simulink model "Mbase4_sim"  (R2014a)
settings: Solver=ode45  StartTime=0.0  StopTime=30  RelTol=1e-3
libraries: arduino_io_lib x5, simulink x1
settings Model: Creator=omar_  LastModifiedBy=omar_

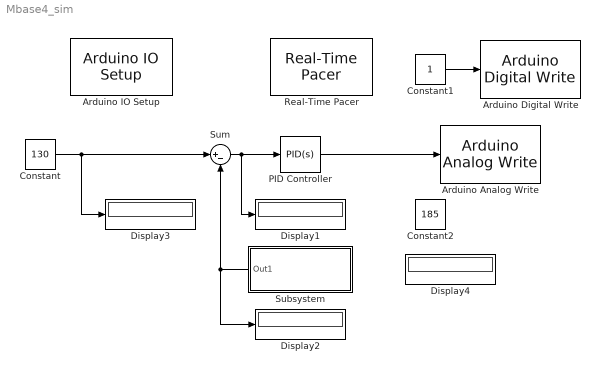
== system Mbase4_sim ==
  Arduino Analog Write : arduino_io_lib/Arduino Analog Write  arduinoVar=Temporary arduino variable: Arduino1  arduinoPin=5  T=0.2
  Arduino Digital Write : arduino_io_lib/Arduino Digital Write  arduinoVar=Temporary arduino variable: Arduino1  arduinoPin=6  T=0.2
  Arduino IO Setup : arduino_io_lib/Arduino IO Setup  Priority=3  arduinoVar=Temporary arduino variable: Arduino1  workspaceVarName=a  comPort=COM3
  Constant : Constant  Value=130
  Constant1 : Constant
  Constant2 : Constant  Value=185
  Display{1..4} (4 alike) : Display
  PID Controller : simulink/Continuous/PID Controller  Controller=PID  TimeDomain=Continuous-time  SampleTime=1  IntegratorMethod=Forward Euler  FilterMethod=Forward Euler  Form=Parallel  P=0.146995673261305  I=0.922603334081805  D=0  N=100  InitialConditionSource=internal  InitialConditionForIntegrator=0  InitialConditionForFilter=0  ExternalReset=none  LimitOutput=off  UpperSaturationLimit=inf  LowerSaturationLimit=-inf  LinearizeAsGain=on  AntiWindupMode=none  Kb=1  TrackingMode=off  Kt=1  PParamMin=[]  PParamMax=[]  IParamMin=[]  IParamMax=[]  DParamMin=[]  DParamMax=[]  NParamMin=[]  NParamMax=[]  KbParamMin=[]  KbParamMax=[]  KtParamMin=[]  KtParamMax=[]  POutMin=[]  POutMax=[]  IOutMin=[]  IOutMax=[]  DOutMin=[]  DOutMax=[]  NOutMin=[]  NOutMax=[]  KbOutMin=[]  KbOutMax=[]  KtOutMin=[]  KtOutMax=[]  IntegratorOutMin=[]  IntegratorOutMax=[]  FilterOutMin=[]  FilterOutMax=[]  SumOutMin=[]  SumOutMax=[]  SumI1OutMin=[]  SumI1OutMax=[]  SumI2OutMin=[]  SumI2OutMax=[]  SumI3OutMin=[]  SumI3OutMax=[]  SumDOutMin=[]  SumDOutMax=[]  SaturationOutMin=[]  SaturationOutMax=[]  IntegratorContinuousStateAttributes=''  IntegratorStateMustResolveToSignalObject=off  IntegratorRTWStateStorageClass=Auto  FilterContinuousStateAttributes=''  FilterStateMustResolveToSignalObject=off  FilterRTWStateStorageClass=Auto
  Real-Time Pacer : arduino_io_lib/Real-Time Pacer  simTimePerRealTime=1
  Subsystem : Subsystem
  Sum : Sum  Inputs=|+-
  wires:
  Constant/1 -> Sum/1, Display3/1
  Sum/1 -> PID Controller/1, Display1/1
  Subsystem/1(Out1) -> Display2/1, Sum/2
  PID Controller/1 -> Arduino Analog Write/1
  Constant1/1 -> Arduino Digital Write/1

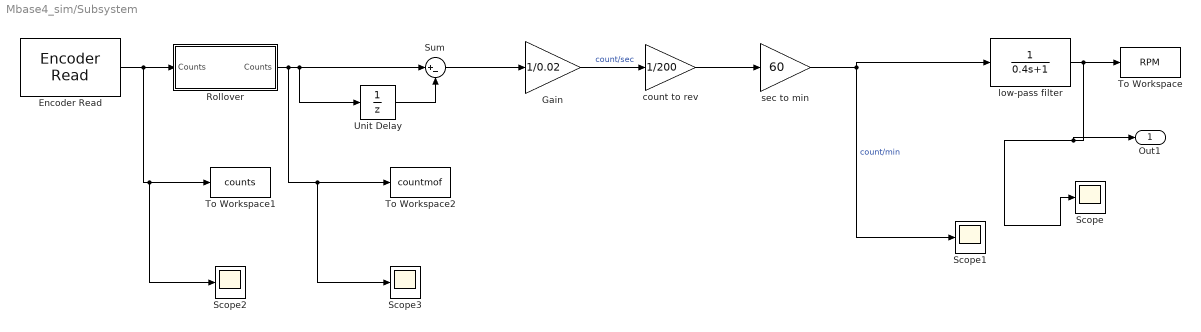
== system Mbase4_sim/Subsystem ==
  Encoder Read : arduino_io_lib/Encoder Read  arduinoVar=Temporary arduino variable: Arduino1  encNum=0  pinA=19  pinB=20  DbDl=0  T=0.02
  Gain : Gain  Gain=1/0.02
  Rollover : Subsystem
  Scope{,1..3} (4 alike) : Scope
      Scope settings: TimeRange=10  YMin=125  YMax=152.5  Decimation=3
      Scope1 settings: TimeRange=30  YMin=-800  YMax=800  Decimation=3
      Scope2 settings: TimeRange=30  YMin=172.9  YMax=191.1  SaveName=ScopeData2  Decimation=3
      Scope3 settings: TimeRange=30  YMin=0  YMax=25000  SaveName=ScopeData3  Decimation=3
  Sum : Sum  Inputs=|+-
  To Workspace : ToWorkspace  VariableName=RPM  SampleTime=-1
  To Workspace1 : ToWorkspace  VariableName=counts  SampleTime=-1
      settings: Save2DSignal=2-D array (concatenate along first dimension)
  To Workspace2 : ToWorkspace  VariableName=countmof  SampleTime=-1
      settings: Save2DSignal=2-D array (concatenate along first dimension)
  Unit Delay : UnitDelay  SampleTime=-1
  count to rev : Gain  Gain=1/200
  low-pass filter : TransferFcn  Denominator=[0.4 1]
  sec to min : Gain  Gain=60
  Out1 : Outport
  wires:
  sec to min/1 -> low-pass filter/1, Scope1/1  "count/min"
  low-pass filter/1 -> Out1/1, Scope/1, To Workspace/1
  Unit Delay/1 -> Sum/2
  Sum/1 -> Gain/1
  Gain/1 -> count to rev/1  "count/sec"
  count to rev/1 -> sec to min/1
  Encoder Read/1 -> Scope2/1, To Workspace1/1, Rollover/1(Counts)
  Rollover/1("Counts ") -> Scope3/1, To Workspace2/1, Unit Delay/1, Sum/1

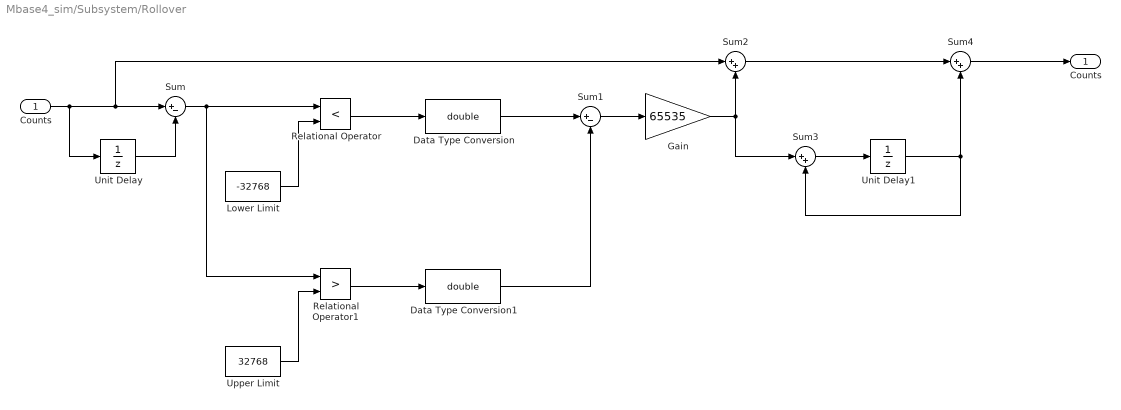
== system Mbase4_sim/Subsystem/Rollover ==
  Counts : Inport
  Data Type Conversion : DataTypeConversion  OutDataTypeStr=double  RndMeth=Zero
  Data Type Conversion1 : DataTypeConversion  OutDataTypeStr=double  RndMeth=Zero
  Gain : Gain  Gain=65535
  Lower Limit : Constant  Value=-32768
  Relational Operator : RelationalOperator  Operator=<  OutDataTypeStr=boolean
  Relational Operator1 : RelationalOperator  Operator=>  OutDataTypeStr=boolean
  Sum : Sum  Inputs=|+-
  Sum1 : Sum  Inputs=|+-
  Sum2 : Sum  Inputs=|++
  Sum3 : Sum  Inputs=|++
  Sum4 : Sum  Inputs=|++
  Unit Delay : UnitDelay  SampleTime=-1
  Unit Delay1 : UnitDelay  SampleTime=-1
  Upper Limit : Constant  Value=32768
  "Counts " : Outport
  wires:
  Counts/1 -> Unit Delay/1, Sum2/1, Sum/1
  Unit Delay/1 -> Sum/2
  Sum/1 -> Relational Operator/1, Relational Operator1/1
  Lower Limit/1 -> Relational Operator/2
  Upper Limit/1 -> Relational Operator1/2
  Relational Operator/1 -> Data Type Conversion/1
  Relational Operator1/1 -> Data Type Conversion1/1
  Data Type Conversion1/1 -> Sum1/2
  Data Type Conversion/1 -> Sum1/1
  Sum1/1 -> Gain/1
  Gain/1 -> Sum3/1, Sum2/2
  Sum4/1 -> "Counts "/1
  Sum2/1 -> Sum4/1
  Sum3/1 -> Unit Delay1/1
  Unit Delay1/1 -> Sum4/2, Sum3/2
